simulink model "sevenstatemodel"  (R2020b)
settings: Solver=VariableStepAuto  StartTime=0.0  StopTime=10  RelTol=1e-3
values from neighbouring files (symbols this model uses):
  Beq = 0.2963    [milestone1constants.m]
  il_i = 0.4    [milestone1constants.m]
  ir_i = 0.4    [milestone1constants.m]
  Jeq = 0.01802    [milestone1constants.m]
  Kb = 2.2179e-3    (= 0.0022179)    [milestone1constants.m]
  Keq = 0.74    [milestone1constants.m]
  la = 0.002    [milestone1constants.m]
  Nmotor = 333.6375    [milestone1constants.m]
  p = 0.037    [milestone1constants.m]
  ra = 7.4    [milestone1constants.m]
  step_time = 5    [milestone1constants.m]
  theta_i = 0    [milestone1constants.m]
  u_l_f = 3    [milestone1constants.m]
  u_l_i = 5    [milestone1constants.m]
  u_r_f = 9    [milestone1constants.m]
  u_r_i = 10    [milestone1constants.m]
  Wr = 0.18    [milestone1constants.m]
  wr_i = 0    [milestone1constants.m]
  x_i = 0    [milestone1constants.m]
  y_i = 0    [milestone1constants.m]
settings Model: Creator=oliviaball  LastModifiedBy=oliviaball
settings DataIOCC: ReturnWorkspaceOutputs=off
settings DebuggingCC: ArithmeticOperatorsInVariantConditions=warning
settings SFSimCC: CustomCodeUndefinedFunction=UseInterfaceOnly

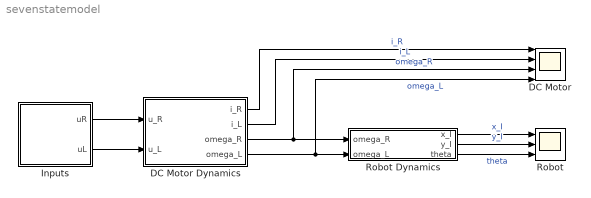
== system sevenstatemodel ==
  DC Motor : Scope  NumInputPorts=4
  DC Motor Dynamics : Subsystem
  Inputs : Subsystem
  "Robot " : Scope  NumInputPorts=3
  Robot Dynamics : Subsystem
  wires:
  DC Motor Dynamics/3(omega_R) -> Robot Dynamics/1(omega_R), DC Motor/3  "omega_R"
  DC Motor Dynamics/4(omega_L) -> DC Motor/4, Robot Dynamics/2(omega_L)  "omega_L"
  Robot Dynamics/2("y_I ") -> "Robot "/2  "y_I"
  Robot Dynamics/3(theta) -> "Robot "/3  "theta"
  Robot Dynamics/1(x_I) -> "Robot "/1  "x_I"
  DC Motor Dynamics/1(i_R) -> DC Motor/1  "i_R"
  DC Motor Dynamics/2(i_L) -> DC Motor/2  "i_L"
  Inputs/1(uR) -> DC Motor Dynamics/1(u_R)
  Inputs/2(uL) -> DC Motor Dynamics/2(u_L)

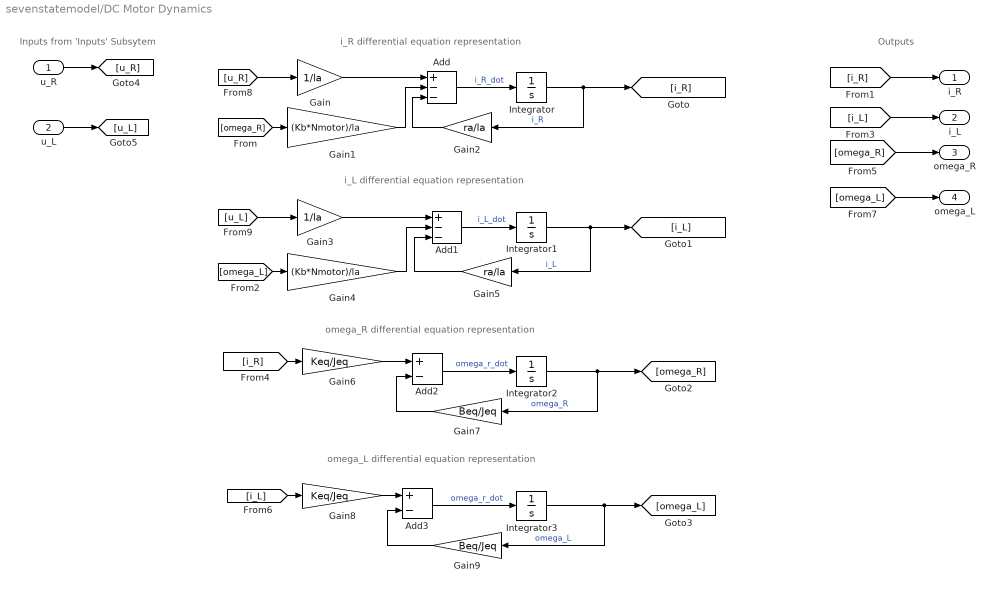
== system sevenstatemodel/DC Motor Dynamics ==
  note: Inputs from 'Inputs' Subsytem
  note: omega_L differential equation representation
  note: omega_R differential equation representation
  note: i_L differential equation representation
  note: i_R differential equation representation
  note: Outputs
  u_R : Inport
  u_L : Inport  Port=2
  Add : Sum  Inputs=+--
  Add1 : Sum  Inputs=+--
  Add2 : Sum  Inputs=+-
  Add3 : Sum  Inputs=+-
  Gain : Gain  Gain=1/la
  Gain1 : Gain  Gain=(Kb*Nmotor)/la
  Gain2 : Gain  Gain=ra/la
  Gain3 : Gain  Gain=1/la
  Gain4 : Gain  Gain=(Kb*Nmotor)/la
  Gain5 : Gain  Gain=ra/la
  Gain6 : Gain  Gain=Keq/Jeq
  Gain7 : Gain  Gain=Beq/Jeq
  Gain8 : Gain  Gain=Keq/Jeq
  Gain9 : Gain  Gain=Beq/Jeq
  Integrator : Integrator  InitialCondition=ir_i
  Integrator1 : Integrator  InitialCondition=il_i
  Integrator2 : Integrator  InitialCondition=wr_i
  Integrator3 : Integrator  InitialCondition=wr_i
  i_R : Outport  VectorParamsAs1DForOutWhenUnconnected=off
  i_L : Outport  Port=2  VectorParamsAs1DForOutWhenUnconnected=off
  omega_R : Outport  Port=3  VectorParamsAs1DForOutWhenUnconnected=off
  omega_L : Outport  Port=4  VectorParamsAs1DForOutWhenUnconnected=off
  wires:
  [u_R] -> Gain/1
  Gain/1 -> Add/1
  [omega_R] -> Gain1/1
  Gain1/1 -> Add/2
  Add/1 -> Integrator/1  "i_R_dot"
  Integrator/1 -> Gain2/1, [i_R]  "i_R"
  Gain2/1 -> Add/3
  Integrator1/1 -> [i_L], Gain5/1  "i_L"
  Gain4/1 -> Add1/2
  Add1/1 -> Integrator1/1  "i_L_dot"
  Gain3/1 -> Add1/1
  [omega_L] -> Gain4/1
  [u_L] -> Gain3/1
  Gain5/1 -> Add1/3
  [i_R] -> Gain6/1
  Gain6/1 -> Add2/1
  Gain7/1 -> Add2/2
  Add2/1 -> Integrator2/1  "omega_r_dot"
  Integrator2/1 -> Gain7/1, [omega_R]  "omega_R"
  [omega_R] -> omega_R/1
  [i_L] -> Gain8/1
  Gain9/1 -> Add3/2
  Add3/1 -> Integrator3/1  "omega_r_dot"
  Integrator3/1 -> Gain9/1, [omega_L]  "omega_L"
  Gain8/1 -> Add3/1
  [omega_L] -> omega_L/1
  [i_L] -> i_L/1
  [i_R] -> i_R/1
  u_R/1 -> [u_R]
  u_L/1 -> [u_L]

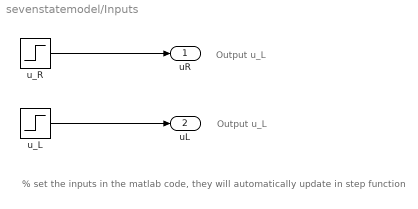
== system sevenstatemodel/Inputs ==
  note: Output u_L
  note: Output u_L
  note: % set the inputs in the matlab code, they will automatically update in step function
  u_L : Step  Time=step_time  Before=u_l_i  After=u_l_f  SampleTime=0
  u_R : Step  Time=step_time  Before=u_r_i  After=u_r_f  SampleTime=0
  uR : Outport  VectorParamsAs1DForOutWhenUnconnected=off
  uL : Outport  Port=2  VectorParamsAs1DForOutWhenUnconnected=off
  wires:
  u_R/1 -> uR/1
  u_L/1 -> uL/1

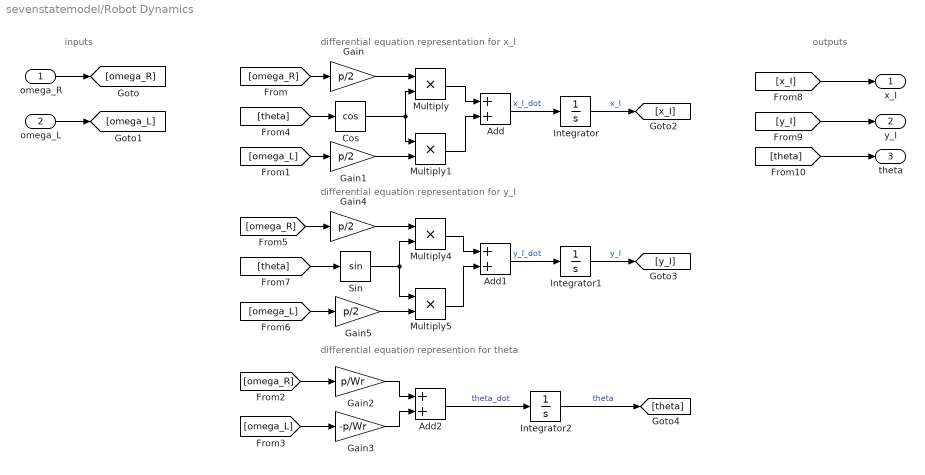
== system sevenstatemodel/Robot Dynamics ==
  note: differential equation represention for theta
  note: outputs
  note: differential equation representation for x_I
  note: inputs
  note: differential equation representation for y_I
  omega_R : Inport
  omega_L : Inport  Port=2
  Add : Sum
  Add1 : Sum
  Add2 : Sum
  Cos : Trigonometry  Operator=cos
  Gain{,1,4..5} (4 alike) : Gain  Gain=p/2
  Gain2 : Gain  Gain=p/Wr
  Gain3 : Gain  Gain=-p/Wr
  Integrator : Integrator  InitialCondition=y_i
  Integrator1 : Integrator  InitialCondition=x_i
  Integrator2 : Integrator  InitialCondition=theta_i
  Multiply{,1,4..5} (4 alike) : Product
  Sin : Trigonometry
  x_I : Outport  VectorParamsAs1DForOutWhenUnconnected=off
  "y_I " : Outport  Port=2  VectorParamsAs1DForOutWhenUnconnected=off
  theta : Outport  Port=3  VectorParamsAs1DForOutWhenUnconnected=off
  wires:
  omega_R/1 -> [omega_R]
  omega_L/1 -> [omega_L]
  [omega_R] -> Gain/1
  [omega_L] -> Gain1/1
  [theta] -> Cos/1
  Cos/1 -> Multiply1/1, Multiply/2
  Gain1/1 -> Multiply1/2
  Gain/1 -> Multiply/1
  Multiply/1 -> Add/1
  Multiply1/1 -> Add/2
  Add/1 -> Integrator/1  "x_I_dot"
  Integrator/1 -> [x_I]  "x_I"
  [theta] -> Sin/1
  Multiply5/1 -> Add1/2
  [omega_R] -> Gain4/1
  [omega_L] -> Gain5/1
  Add1/1 -> Integrator1/1  "y_I_dot"
  Integrator1/1 -> [y_I]  "y_I"
  Gain4/1 -> Multiply4/1
  Sin/1 -> Multiply5/1, Multiply4/2
  Multiply4/1 -> Add1/1
  [omega_R] -> Gain2/1
  Gain2/1 -> Add2/1
  [omega_L] -> Gain3/1
  Gain3/1 -> Add2/2
  Add2/1 -> Integrator2/1  "theta_dot"
  Integrator2/1 -> [theta]  "theta"
  [x_I] -> x_I/1
  [y_I] -> "y_I "/1
  [theta] -> theta/1
  Gain5/1 -> Multiply5/2
